simulink model "Simulink_Observation_5"  (R2020b)
settings: Solver=VariableStepAuto  StartTime=0.0  StopTime=0  RelTol=1e-3
settings Model: Creator=Mohit Akhouri  LastModifiedBy=Mohit Akhouri

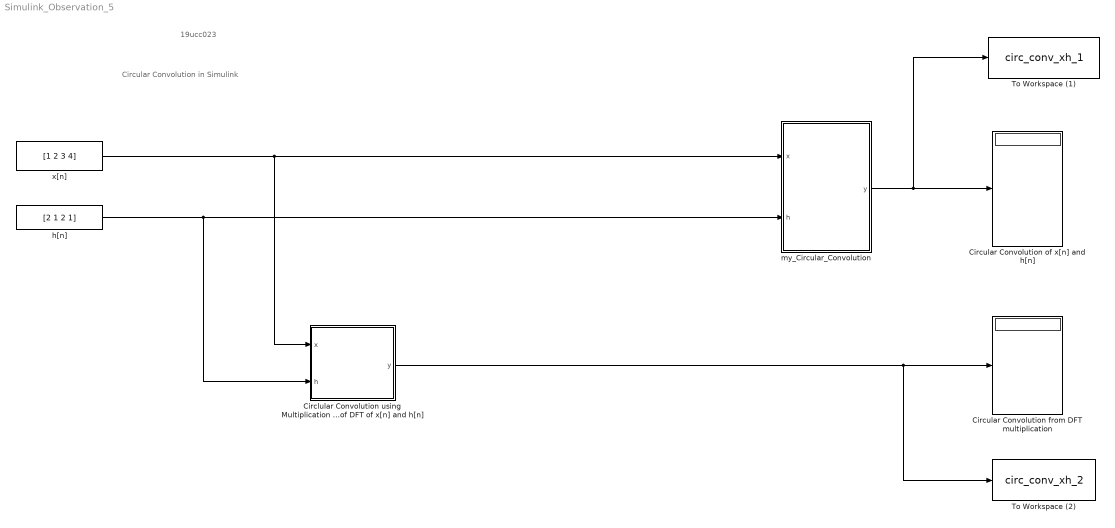
== system Simulink_Observation_5 ==
  note: Circular Convolution in Simulink
  note: 19ucc023
  Circlular Convolution using Multiplication of DFT of x[n] and h[n] : MATLAB Function  TreatAsAtomicUnit=on
  Circular Convolution from DFT multiplication : Display
  Circular Convolution of x[n] and h[n] : Display
  To Workspace (1) : ToWorkspace  VariableName=circ_conv_xh_1  SaveFormat=Timeseries  SampleTime=-1
  To Workspace (2) : ToWorkspace  VariableName=circ_conv_xh_2  SaveFormat=Timeseries  SampleTime=-1
  h[n] : Constant  Value=[2 1 2 1]
  my_Circular_Convolution : MATLAB Function  TreatAsAtomicUnit=on
  x[n] : Constant  Value=[1 2 3 4]
  wires:
  h[n]/1 -> Circlular Convolution using Multiplication of DFT of x[n] and h[n]/2(h), my_Circular_Convolution/2(h)
  x[n]/1 -> Circlular Convolution using Multiplication of DFT of x[n] and h[n]/1(x), my_Circular_Convolution/1(x)
  my_Circular_Convolution/1(y) -> To Workspace (1)/1, Circular Convolution of x[n] and h[n]/1
  Circlular Convolution using Multiplication of DFT of x[n] and h[n]/1(y) -> To Workspace (2)/1, Circular Convolution from DFT multiplication/1

== matlab function Simulink_Observation_5/Circlular Convolution using Multiplication of DFT of x[n] and h[n] ==
  data: x input; y output; h input
function y = fcn(x,h)

X = fft(x,4);
H = fft(h,4);
Y = X .* H;
y = abs(ifft(Y,4));

== matlab function Simulink_Observation_5/my_Circular_Convolution ==
  data: x input; y output; h input
function y = fcn(x,h)
% This function will calculate the circular convolution 
% of input sequence x[n] and impulse response h[n]

% 19ucc023 
% Mohit Akhouri

% ALGORITHM : First make the length of both sequences equal , then call
% myCirConvMat function to calculate the circular convolution matrix.
% Now multiply the Matrix with 'column-vector' x[n] to get the final result

% Making the length of the two sequences equal by 'PADDING WITH ZEROS'

length_x = length(x); % length of input sequence x[n]
length_h = length(h); % length of impulse response h[n]

if(length_x > length_h)
    h = [h zeros(1,length_x - length_h)]; % padding 'h[n]' with zeros
    length_h = length(h);
else
    x = [x zeros(1,length_h - length_x)]; % padding 'x[n]' with zeros
    length_x = length(x);
end

n = length_x; % length of input sequence x[n] to be passed to function

% Calling the myCirConvMat function to calculate the circular convolution
% matrix and storing it in variable H

H = myCirConvMat(h,n); % calling the function for Circular Conv. matrix

% Algorithm for calculation of circular convolution is as follows

y = zeros(1,n); % initializing the output vector 

for i=1:n
    sum = 0;
    for j=1:n
       sum = sum + (H(i,j)*x(j));
    end
    y(i) = sum;
end

end
